simulink model "y002"  (R2019b)
settings: Solver=ode23tb  StartTime=0.0  StopTime=1  RelTol=1e-3
values from neighbouring files (symbols this model uses):
  fN = 50    [parameter.m]
  J = 0.1284    [parameter.m]
  Llr = Lr - Lm    (= 0.006)    [parameter.m]
  Lls = Ls - Lm    (= 0.0102)    [parameter.m]
  np = 2    [parameter.m]
  PN = 3000    [parameter.m]
  Rr = 2.685    [parameter.m]
  Rs = 1.85    [parameter.m]
  TN = PN/(2*pi*nN/60)    (= 20.4627783975)    [parameter.m]
  UN = 380    [parameter.m]
undefined symbols (not defined in the file or in its folder): i
libraries: powerlib x5, simulink x1
Description:
  | Clarke\Park正反变换测试
settings Model: Creator=Inspiron  LastModifiedBy=Inspiron

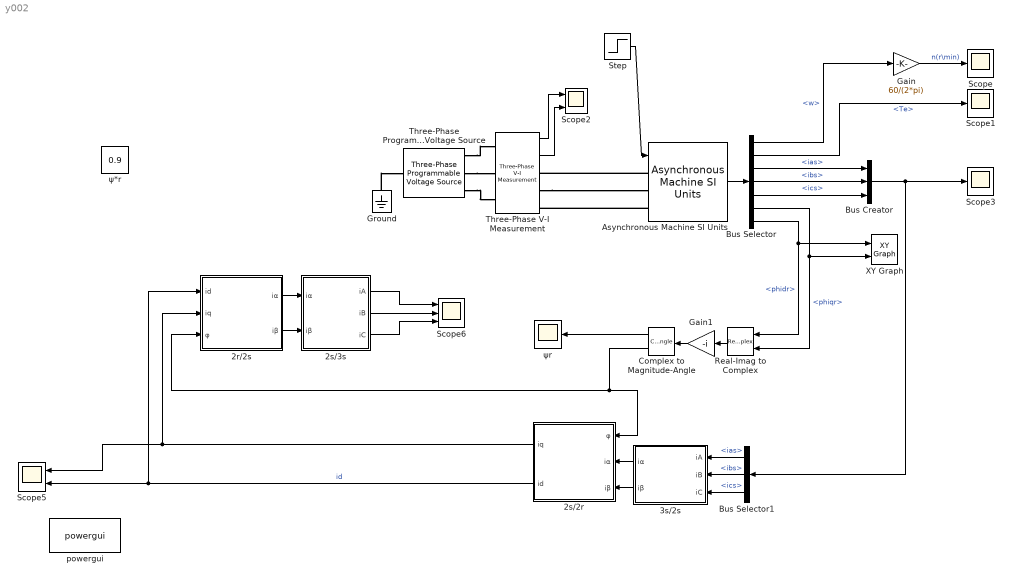
== system y002 ==
  2r/2s : Subsystem
  2s/2r : Subsystem
  2s/3s : Subsystem
  3s/2s : Subsystem
  Asynchronous Machine SI Units : powerlib/Machines/Asynchronous Machine SI Units  RotorType=Squirrel-cage  PresetModel=No  MechanicalLoad=Torque Tm  ShowDetailedParameters=on  ReferenceFrame=Stationary  Units=SI  MeasurementBus=on  NominalParameters=[PN UN fN]  Stator=[Rs Lls]  Rotor=[Rr Llr]  Cage1=[0.4155 0.002066]  Cage2=[0.4168 0.0003495]  Lm=Lm  Mechanical=[J 0 np]  PolePairs=2  InitialConditions=[1 0 0 0 0 0 0 0]  SimulateSaturation=off  Saturation=[14.03593122, 27.81365428, 53.79336849, 72.68890987, 97.98006896, 148.6815601, 215.7428561, 302.9841135, 428.7778367 ; 230, 322, 414, 460, 506, 552, 598, 644, 690]  LoadFlowParameters=1492000  TsPowergui=0  TsBlock=-1  IterativeModel=Trapezoidal non iterative  IterativeDiscreteModel=Trapezoidal non iterative  Pmec=1.492e+006
      settings: SourceProductName=Simscape Electrical
  Bus Creator : BusCreator  Inputs=3
  Bus Selector : BusSelector  OutputSignals=w,Te,ias,ibs,ics,phiqr,phidr
  Bus Selector1 : BusSelector  OutputSignals=ias,ibs,ics
  Complex to Magnitude-Angle : ComplexToMagnitudeAngle
  Gain : Gain  Gain=60/(2*pi)
  Gain1 : Gain  Gain=-i
  Ground : powerlib/Elements/Ground  LConnTagsString=a
      settings: SourceProductName=Simscape Electrical
  Real-Imag to Complex : RealImagToComplex
  Scope : Scope
  Scope1 : Scope
  Scope2 : Scope  NumInputPorts=2
  Scope3 : Scope
  Scope5 : Scope  NumInputPorts=2
  Scope6 : Scope  NumInputPorts=3
  Step : Step  Time=0.7  After=TN  VectorParams1D=off  ZeroCross=off
  Three-Phase Programmable Voltage Source : powerlib/Electrical Sources/Three-Phase Programmable Voltage Source  PositiveSequence="[380  0 50]"  VariationEntity=None  VariationType=Table of time-amplitude pairs  VariationTypeAlt=Step  VariationStep=0.5  VariationRate=10  VariationMagnitude=0.3  VariationFrequency=2  VariationTiming=[1 2]  VariationPhaseA=off  Amplitudes=[1 0.8 1.2 1.0]  TimeValues=[0 0.1 0.15 0.2]  HarmonicGeneration=off  HarmonicA=[3 0.2 -25 0]  HarmonicB=[2 0.15 35 2]  Timing="[0.05  3]"  BusType=swing  Pref=0  Qref=0  Qmin=-inf  Qmax=inf
      settings: SourceProductName=Simscape Electrical
  Three-Phase V-I Measurement : powerlib/Measurements/Three-Phase V-I Measurement  VoltageMeasurement=phase-to-ground  SetLabelV=off  LabelV=Vabc  Vpu=off  VpuLL=off  CurrentMeasurement=yes  SetLabelI=off  LabelI=Iabc  Ipu=off  Pbase=100e6  Vbase=500e3  OutputType=Complex  PhasorSimulation=off  PSBequivalent=0
      settings: SourceProductName=Simscape Electrical
  XY Graph : simulink/Sinks/XY Graph  xmin=-1  xmax=1  ymin=-1  ymax=1  st=-1
  powergui : powerlib/powergui  Priority=1  SimulationMode=Continuous  SampleTime=50e-6  frequency=60  Iterations=50  frequencyindice=50  Pbase=100e6  ErrMax=1e-4  UnitsV=kV  UnitsW=MW  buscounter=0  FunctionMessages=off  echomessages=off  EnableUseOfTLC=off  CurrentSourceSwitches=off  DisableSnubberDevices=off  DisableRonSwitches=off  DisableVfSwitches=off  DisplayEquations=off  AutomaticDiscreteSolvers=off  SolverType=Tustin/Backward Euler (TBE)  Interpol=off  ExternalGateDelay=off  methode=off  Ts=100  x0status=blocks  SPID=on  SwTol=0  HookPort=off  NonlinearTolerance=1e-4  nMaxIteration=100  ContinueOnMaxIteration=off  RestoreLinks=warning  ResistiveCurrentMeasurement=off  Frange=[0:2:500]  Ylog=off  Xlog=on  ShowGrid=off  save=off  variable=ZData  structure=0  ZoomFFT=off  StartTime=0.0  cycles=1  DisplayStyle=1  fundamental=60  FreqAxis=off  MaxFrequency=1000  frequencyindicesteady=1  RmsSteady=1  display=off
      settings: SourceProductName=Simscape Electrical
  ψ*r : Constant  Value=0.9
  ψr : Scope
  wires:
  Asynchronous Machine SI Units/1 -> Bus Selector/1
  Step/1 -> Asynchronous Machine SI Units/1
  Three-Phase V-I Measurement/1 -> Scope2/1
  Three-Phase V-I Measurement/2 -> Scope2/2
  Bus Creator/1 -> Bus Selector1/1, Scope3/1
  Gain/1 -> Scope/1  "n(r\\min)"
  Bus Selector1/1 -> 3s/2s/1(iA)  "<ias>"
  Bus Selector1/2 -> 3s/2s/2(iB)  "<ibs>"
  Bus Selector1/3 -> 3s/2s/3(iC)  "<ics>"
  Bus Selector/1 -> Gain/1  "<w>"
  Bus Selector/2 -> Scope1/1  "<Te>"
  Bus Selector/3 -> Bus Creator/1  "<ias>"
  Bus Selector/4 -> Bus Creator/2  "<ibs>"
  Bus Selector/5 -> Bus Creator/3  "<ics>"
  3s/2s/1(iα) -> 2s/2r/2(iα)
  3s/2s/2(iβ) -> 2s/2r/3(iβ)
  Real-Imag to Complex/1 -> Gain1/1
  Bus Selector/6 -> XY Graph/2, Real-Imag to Complex/2  "<phiqr>"
  Bus Selector/7 -> XY Graph/1, Real-Imag to Complex/1  "<phidr>"
  Complex to Magnitude-Angle/2 -> 2s/2r/1(φ), 2r/2s/3(φ)
  2s/2r/2(id) -> 2r/2s/1(id), Scope5/2  "id"
  2s/2r/1(iq) -> 2r/2s/2(iq), Scope5/1
  Complex to Magnitude-Angle/1 -> ψr/1
  2r/2s/1(iα) -> 2s/3s/1(iα)
  2r/2s/2(iβ) -> 2s/3s/2(iβ)
  2s/3s/1(iA) -> Scope6/1
  2s/3s/3(iC) -> Scope6/3
  2s/3s/2(iB) -> Scope6/2
  Gain1/1 -> Complex to Magnitude-Angle/1
  connections:
  Three-Phase Programmable Voltage Source/RConn1 -- Three-Phase V-I Measurement/LConn1
  Three-Phase Programmable Voltage Source/RConn2 -- Three-Phase V-I Measurement/LConn2
  Three-Phase Programmable Voltage Source/RConn3 -- Three-Phase V-I Measurement/LConn3
  Asynchronous Machine SI Units/LConn1 -- Three-Phase V-I Measurement/RConn1
  Three-Phase V-I Measurement/RConn2 -- Asynchronous Machine SI Units/LConn2
  Asynchronous Machine SI Units/LConn3 -- Three-Phase V-I Measurement/RConn3
  Ground/LConn1 -- Three-Phase Programmable Voltage Source/LConn1

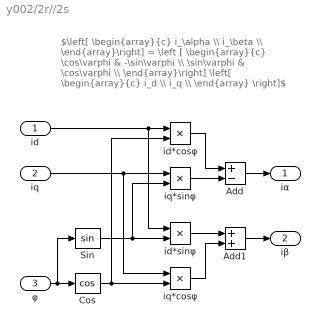
== system y002/2r//2s ==
  note: $\left[ \begin{array}{c} i_\alpha \\ i_\beta \\ \end{array}\right] = \left [ \begin{array}{c} \cos\varphi & -\sin\varphi \\ \sin\varphi & \cos\varphi \\ \end{array}\right] \left[ \begin{array}{c} i_d \\ i_q \\ \end{array} \right]$
  id : Inport
  iq : Inport  Port=2
  φ : Inport  Port=3
  Add : Sum  Inputs=+-
  Add1 : Sum
  Cos : Trigonometry  Operator=cos
  Sin : Trigonometry
  id*cosφ : Product
  id*sinφ : Product
  iq*cosφ : Product
  iq*sinφ : Product
  iα : Outport
  iβ : Outport  Port=2
  wires:
  Cos/1 -> iq*cosφ/2, id*cosφ/2
  iq*cosφ/1 -> Add1/2
  Sin/1 -> id*sinφ/2, iq*sinφ/2
  id/1 -> id*cosφ/1, id*sinφ/1
  id*sinφ/1 -> Add1/1
  iq*sinφ/1 -> Add/2
  iq/1 -> iq*sinφ/1, iq*cosφ/1
  φ/1 -> Sin/1, Cos/1
  Add/1 -> iα/1
  id*cosφ/1 -> Add/1
  Add1/1 -> iβ/1

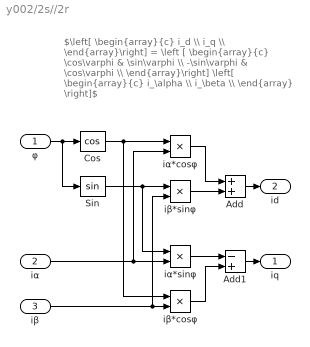
== system y002/2s//2r ==
  note: $\left[ \begin{array}{c} i_d \\ i_q \\ \end{array}\right] = \left [ \begin{array}{c} \cos\varphi & \sin\varphi \\ -\sin\varphi & \cos\varphi \\ \end{array}\right] \left[ \begin{array}{c} i_\alpha \\ i_\beta \\ \end{array} \right]$
  φ : Inport
  iα : Inport  Port=2
  iβ : Inport  Port=3
  Add : Sum
  Add1 : Sum  Inputs=-+
  Cos : Trigonometry  Operator=cos
  Sin : Trigonometry
  iα*cosφ : Product
  iα*sinφ : Product
  iβ*cosφ : Product
  iβ*sinφ : Product
  iq : Outport
  id : Outport  Port=2
  wires:
  Cos/1 -> iα*cosφ/1, iβ*cosφ/1
  iβ*cosφ/1 -> Add1/2
  Sin/1 -> iα*sinφ/1, iβ*sinφ/1
  iα/1 -> iα*sinφ/2, iα*cosφ/2
  iα*sinφ/1 -> Add1/1
  iβ*sinφ/1 -> Add/2
  iβ/1 -> iβ*sinφ/2, iβ*cosφ/2
  φ/1 -> Cos/1, Sin/1
  Add/1 -> id/1
  iα*cosφ/1 -> Add/1
  Add1/1 -> iq/1

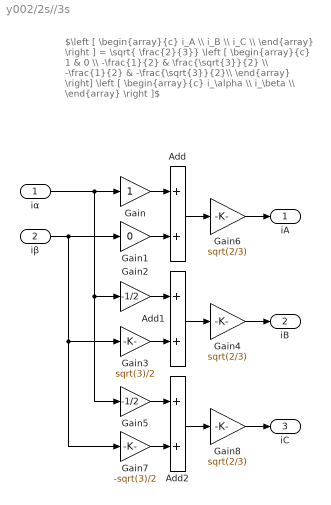
== system y002/2s//3s ==
  note: $\left [ \begin{array}{c} i_A \\ i_B \\ i_C \\ \end{array} \right ] = \sqrt{ \frac{2}{3}} \left [ \begin{array}{c} 1 & 0 \\ -\frac{1}{2} & \frac{\sqrt{3}}{2} \\ -\frac{1}{2} & -\frac{\sqrt{3}}{2}\\ \end{array} \right] \left [ \begin{array}{c} i_\alpha \\ i_\beta \\ \end{array} \right ]$
  iα : Inport
  iβ : Inport  Port=2
  Add : Sum  Inputs=2
  Add1 : Sum  Inputs=2
  Add2 : Sum  Inputs=2
  Gain : Gain
  Gain1 : Gain  Gain=0
  Gain2 : Gain  Gain=-1/2
  Gain3 : Gain  Gain=sqrt(3)/2
  Gain4 : Gain  Gain=sqrt(2/3)
  Gain5 : Gain  Gain=-1/2
  Gain6 : Gain  Gain=sqrt(2/3)
  Gain7 : Gain  Gain=-sqrt(3)/2
  Gain8 : Gain  Gain=sqrt(2/3)
  iA : Outport
  iB : Outport  Port=2
  iC : Outport  Port=3
  wires:
  Gain/1 -> Add/1
  iβ/1 -> Gain7/1, Gain3/1, Gain1/1
  Add/1 -> Gain6/1
  Gain1/1 -> Add/2
  iα/1 -> Gain5/1, Gain2/1, Gain/1
  Gain4/1 -> iB/1
  Gain6/1 -> iA/1
  Gain2/1 -> Add1/1
  Gain3/1 -> Add1/2
  Add1/1 -> Gain4/1
  Gain5/1 -> Add2/1
  Gain7/1 -> Add2/2
  Gain8/1 -> iC/1
  Add2/1 -> Gain8/1

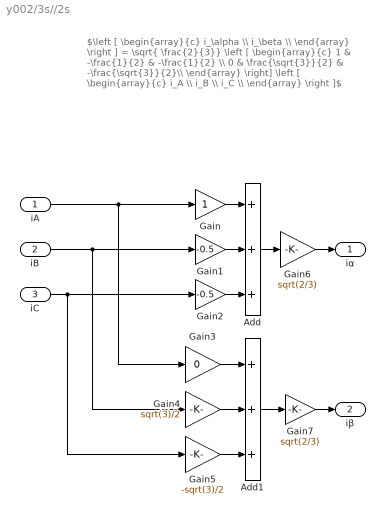
== system y002/3s//2s ==
  note: $\left [ \begin{array}{c} i_\alpha \\ i_\beta \\ \end{array} \right ] = \sqrt{ \frac{2}{3}} \left [ \begin{array}{c} 1 & -\frac{1}{2} & -\frac{1}{2} \\ 0 & \frac{\sqrt{3}}{2} & -\frac{\sqrt{3}}{2}\\ \end{array} \right] \left [ \begin{array}{c} i_A \\ i_B \\ i_C \\ \end{array} \right ]$
  iA : Inport
  iB : Inport  Port=2
  iC : Inport  Port=3
  Add : Sum  Inputs=3
  Add1 : Sum  Inputs=3
  Gain : Gain
  Gain1 : Gain  Gain=-0.5
  Gain2 : Gain  Gain=-0.5
  Gain3 : Gain  Gain=0
  Gain4 : Gain  Gain=sqrt(3)/2
  Gain5 : Gain  Gain=-sqrt(3)/2
  Gain6 : Gain  Gain=sqrt(2/3)
  Gain7 : Gain  Gain=sqrt(2/3)
  iα : Outport
  iβ : Outport  Port=2
  wires:
  Gain4/1 -> Add1/2
  Gain/1 -> Add/1
  Gain5/1 -> Add1/3
  iB/1 -> Gain4/1, Gain1/1
  Add/1 -> Gain6/1
  Gain1/1 -> Add/2
  Gain3/1 -> Add1/1
  iA/1 -> Gain3/1, Gain/1
  Gain2/1 -> Add/3
  iC/1 -> Gain5/1, Gain2/1
  Add1/1 -> Gain7/1
  Gain7/1 -> iβ/1
  Gain6/1 -> iα/1
